simulink model "TA_Plant_Controller_Simulink"  (R2021a)
settings: Solver=ode45  StartTime=0.0  StopTime=1500  RelTol=1e-3  EnableMultiTasking=on
values from neighbouring files (symbols this model uses):
  Acu = 0    [TA_Plant_Controller_Param.m]
  Awa = 0.3    [TA_Plant_Controller_Param.m]
  Awi = 0    [TA_Plant_Controller_Param.m]
  d11 = ((6/11)^2)*d11    (= 74.3801652893)    [TA_Plant_Controller_Param.m]
  d22 = ((6/11)^2)*d22    (= 431.404958678)    [TA_Plant_Controller_Param.m]
  d33 = 10*((6/11)^2)*d33    (= 4314.04958678)    [TA_Plant_Controller_Param.m]
  d44 = ((6/11)^2)*d44    (= 2380.16528926)    [TA_Plant_Controller_Param.m]
  d55 = ((6/11)^2)*d55    (= 44628.0991736)    [TA_Plant_Controller_Param.m]
  d66 = ((6/11)^2)*d66    (= 2380.16528926)    [TA_Plant_Controller_Param.m]
  dp2 = ((6/11)^2)*dp2    (= 0)    [TA_Plant_Controller_Param.m]
  dp3 = 0    [TA_Plant_Controller_Param.m]
  dq2 = ((6/11)^2)*dq2    (= 0)    [TA_Plant_Controller_Param.m]
  dq3 = 0    [TA_Plant_Controller_Param.m]
  dr2 = ((6/11)^2)*dr2    (= 59.5041322314)    [TA_Plant_Controller_Param.m]
  dr3 = 0    [TA_Plant_Controller_Param.m]
  du2 = ((6/11)^2)*du2    (= 59.5041322314)    [TA_Plant_Controller_Param.m]
  du3 = 0    [TA_Plant_Controller_Param.m]
  dv2 = ((6/11)^2)*dv2    (= 273.748760331)    [TA_Plant_Controller_Param.m]
  dv3 = 0    [TA_Plant_Controller_Param.m]
  dw2 = ((6/11)^2)*dw2    (= 273.748760331)    [TA_Plant_Controller_Param.m]
  dw3 = 0    [TA_Plant_Controller_Param.m]
  g = 9.8    [TA_Plant_Controller_Param.m]
  intpitch = 0    [TA_Plant_Controller_Param.m]
  introll = 0    [TA_Plant_Controller_Param.m]
  intz = 0    [TA_Plant_Controller_Param.m]
  Kb = 1000    [TA_Plant_Controller_Param.m]
  kpitch = 50    [TA_Plant_Controller_Param.m]
  kroll = 1.5    [TA_Plant_Controller_Param.m]
  kuu = 1140    [TA_Plant_Controller_Param.m]
  kvr = 20000    [TA_Plant_Controller_Param.m]
  m11 = ((6/11)^2)*m11    (= 312.396694215)    [TA_Plant_Controller_Param.m]
  m22 = ((6/11)^2)*m22    (= 357.024793388)    [TA_Plant_Controller_Param.m]
  m33 = ((6/11)^2)*m33    (= 362.975206612)    [TA_Plant_Controller_Param.m]
  m44 = ((6/11)^2)*m44    (= 459.683676155)    [TA_Plant_Controller_Param.m]
  m55 = ((6/11)^2)*m55    (= 9595.04132231)    [TA_Plant_Controller_Param.m]
  m66 = ((6/11)^2)*m66    (= 9600.99173554)    [TA_Plant_Controller_Param.m]
  mode_gangguan = 1    [TA_Plant_Controller_Param.m]
  rho = 1025    [TA_Plant_Controller_Param.m]
  Ts = 0.05    [TA_Plant_Controller_Param.m]
  vol = ((6/11)^2)*6.6206    (= 1.96976528926)    [TA_Plant_Controller_Param.m]
undefined symbols (not defined in the file or in its folder): magnitude
libraries: mpclib x1, simulink x1
settings Model: Creator=farabialif  LastModifiedBy=billy
settings SolverCC: AlgebraicLoopSolver=TrustRegion
settings DataIOCC: LimitDataPoints=on  SaveFormat=Array  ReturnWorkspaceOutputs=off
settings OptimizationCC: LifeSpan=inf
settings DebuggingCC: SolverPrmCheckMsg=warning  SFUnexpectedBacktrackingDiag=warning  SFNoUnconditionalDefaultTransitionDiag=warning  SFExecutionAtInitializationDiag=none  SFMachineParentedDataDiag=warning  ArithmeticOperatorsInVariantConditions=warning
settings HardwareCC: ProdBitPerPointer=32  ProdBitPerSizeT=32  ProdBitPerPtrDiffT=32  ProdLargestAtomicFloat=None  ProdIntDivRoundTo=Undefined  ProdEndianess=Unspecified  ProdWordSize=32  ProdHWDeviceType=32-bit Generic
settings ModelReferenceCC: PropagateSignalLabelsOutOfModel=off
settings SFSimCC: SimUseLocalCustomCode=off  CustomCodeUndefinedFunction=UseInterfaceOnly
settings RTWCC: RTWUseLocalCustomCode=off
settings CodeAppCC: StateflowObjectComments=on
settings GRTTargetCC: TargetLangStandard=C89/C90 (ANSI)
settings ConfigComp: CovMetricSettings=dw  CovSaveCumulativeToWorkspaceVar=on  CovSaveSingleToWorkspaceVar=on  CovExternalEMLEnable=off  CovSFcnEnable=off

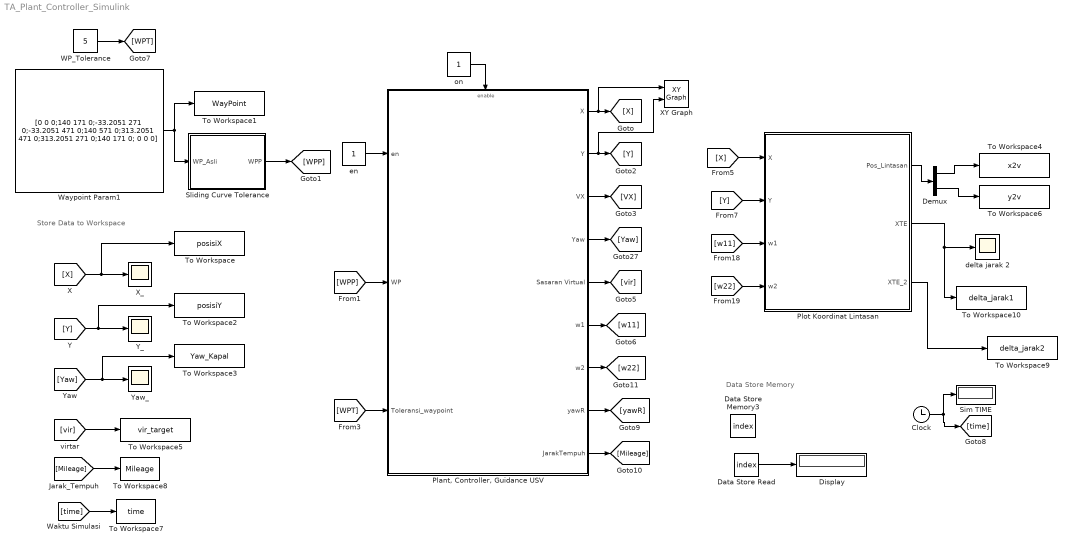
== system TA_Plant_Controller_Simulink ==
  note: Data Store Memory
  note: Store Data to Workspace
  Clock : Clock
  Data Store Memory3 : DataStoreMemory  DataStoreName=index  ReadBeforeWriteMsg=warning  WriteAfterWriteMsg=warning  WriteAfterReadMsg=warning  ShowAdditionalParam=off  OutDataTypeStr=int8  Dimensions=1
  Data Store Read : DataStoreRead  DataStoreName=index  IndexOptions=Index vector (dialog)  Indices=1  OutputSizes=1
  Demux : Demux  Outputs=2
  Display : Display
  "Plant, Controller, Guidance USV" : Subsystem
  Plot Koordinat Lintasan : MATLAB Function  TreatAsAtomicUnit=on
  Sim TIME : Display
  Sliding Curve Tolerance : MATLAB Function  TreatAsAtomicUnit=on
  To Workspace : ToWorkspace  VariableName=posisiX  SaveFormat=Timeseries  SampleTime=-1
  To Workspace1 : ToWorkspace  VariableName=WayPoint  SampleTime=-1
  To Workspace10 : ToWorkspace  VariableName=delta_jarak1  SaveFormat=Timeseries  SampleTime=-1
  To Workspace2 : ToWorkspace  VariableName=posisiY  SaveFormat=Timeseries  SampleTime=-1
  To Workspace3 : ToWorkspace  VariableName=Yaw_Kapal  SaveFormat=Timeseries  SampleTime=-1
  To Workspace4 : ToWorkspace  VariableName=x2v  SaveFormat=Timeseries  SampleTime=-1
  To Workspace5 : ToWorkspace  VariableName=vir_target  SaveFormat=Timeseries  SampleTime=-1
  To Workspace6 : ToWorkspace  VariableName=y2v  SaveFormat=Timeseries  SampleTime=-1
  To Workspace7 : ToWorkspace  VariableName=time  SaveFormat=Timeseries  SampleTime=-1
  To Workspace8 : ToWorkspace  VariableName=Mileage  SaveFormat=Timeseries  SampleTime=-1
  To Workspace9 : ToWorkspace  VariableName=delta_jarak2  SaveFormat=Timeseries  SampleTime=-1
  WP_Tolerance : Constant  Value=5
  Waypoint Param1 : Constant  Value=[0 0 0;140 171 0;-33.2051 271 0;-33.2051 471 0;140 571 0;313.2051 471 0;313.2051 271 0;140 171 0; 0 0 0]
  XY Graph : simulink/Sinks/XY Graph  xmin=-100  xmax=350  ymin=-20  ymax=600  st=-1
  X_ : Scope
  Y_ : Scope
  Yaw_ : Scope
  delta jarak 2 : Scope
  en : Constant
  on : Constant
  wires:
  on/1 -> "Plant, Controller, Guidance USV"/Enable
  en/1 -> "Plant, Controller, Guidance USV"/1("en ")
  WP_Tolerance/1 -> [WPT]
  [WPT] -> "Plant, Controller, Guidance USV"/3(Toleransi_waypoint)
  [Y] -> To Workspace2/1, Y_/1
  [X] -> To Workspace/1, X_/1
  [Yaw] -> To Workspace3/1, Yaw_/1
  [vir] -> To Workspace5/1
  Waypoint Param1/1 -> Sliding Curve Tolerance/1(WP_Asli), To Workspace1/1
  [WPP] -> "Plant, Controller, Guidance USV"/2(WP)
  "Plant, Controller, Guidance USV"/6(w1) -> [w11]
  "Plant, Controller, Guidance USV"/1(X) -> XY Graph/1, [X]
  "Plant, Controller, Guidance USV"/2(Y) -> XY Graph/2, [Y]
  "Plant, Controller, Guidance USV"/5(Sasaran Virtual) -> [vir]
  "Plant, Controller, Guidance USV"/4(Yaw) -> [Yaw]
  "Plant, Controller, Guidance USV"/7(w2) -> [w22]
  "Plant, Controller, Guidance USV"/3(VX) -> [VX]
  [X] -> Plot Koordinat Lintasan/1(X)
  [Y] -> Plot Koordinat Lintasan/2(Y)
  [w11] -> Plot Koordinat Lintasan/3(w1)
  [w22] -> Plot Koordinat Lintasan/4(w2)
  Clock/1 -> [time], Sim TIME/1
  "Plant, Controller, Guidance USV"/8(yawR) -> [yawR]
  "Plant, Controller, Guidance USV"/9(JarakTempuh) -> [Mileage]
  Data Store Read/1 -> Display/1
  Sliding Curve Tolerance/1(WPP) -> [WPP]
  Plot Koordinat Lintasan/1(Pos_Lintasan) -> Demux/1
  Demux/1 -> To Workspace4/1
  Demux/2 -> To Workspace6/1
  Plot Koordinat Lintasan/2(XTE) -> To Workspace10/1, delta jarak 2/1
  [Mileage] -> To Workspace8/1
  [time] -> To Workspace7/1
  Plot Koordinat Lintasan/3(XTE_2) -> To Workspace9/1

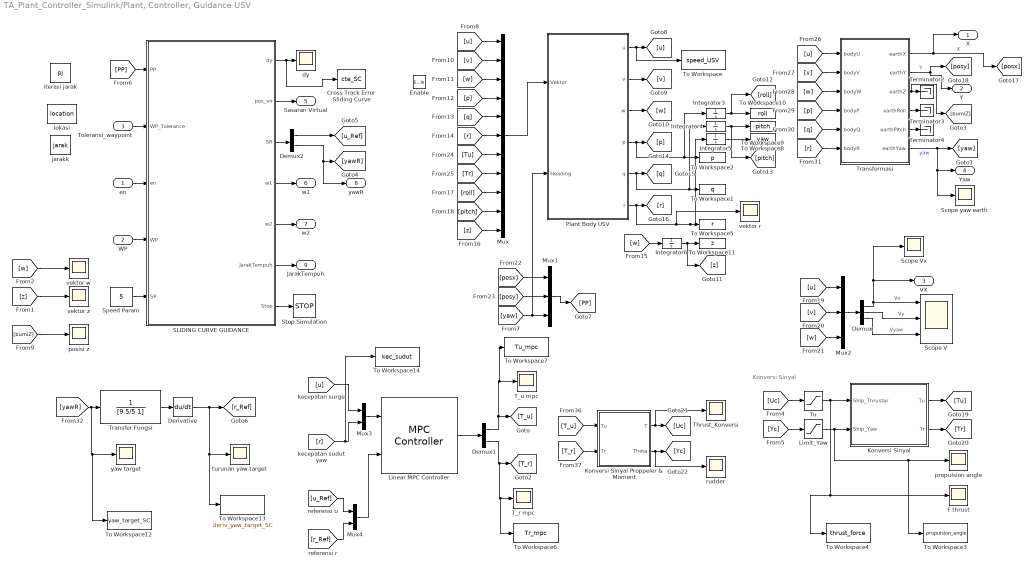
== system TA_Plant_Controller_Simulink/Plant, Controller, Guidance USV ==
  note: Konversi Sinyal
  "en " : Inport
  WP : Inport  Port=2
  Toleransi_waypoint : Inport  Port=3
  Enable : EnablePort
  Cross Track Error Sliding Curve : ToWorkspace  VariableName=cte_SC  SaveFormat=Timeseries  SampleTime=Ts
  Demux : Demux  Outputs=3
  Demux1 : Demux  Outputs=2
  Demux2 : Demux  Outputs=2
  Derivative : Derivative  CoefficientInTFapproximation=Ts
  F thrust : Scope
  Integrator3 : Integrator  InitialCondition=introll
  Integrator4 : Integrator  InitialCondition=intpitch
  Integrator5 : Integrator
  Integrator6 : Integrator  InitialCondition=intz
  Konversi Sinyal : MATLAB Function  TreatAsAtomicUnit=on
  Konversi Sinyal Proppeler & Moment : MATLAB Function  TreatAsAtomicUnit=on
  Limit_Yaw : Saturate  UpperLimit=1.0472  LowerLimit=-1.0472
  Linear MPC Controller : mpclib/MPC Controller  SCDEnableBlockLinearizationSpecification=on  mpcobj=mpc04  is_multiple=0  enable_value=0  return_u0=off  updateMPCinCallerWorkspace=on  md_inport=off  mv_inport=off  uref_inport=off  return_cost=off  return_mvseq=off  return_qpstatus=off  return_xseq=off  return_state=off  return_ovseq=off  state_inport=off  umin_inport=off  umax_inport=off  ymin_inport=off  ymax_inport=off  cc_inport=off  ywt_inport=off  uwt_inport=off  duwt_inport=off  rhoeps_inport=off  pm_inport=off  MaximumP=10  HorizonChoice=FixedHorizon  n_ts=0.05  n_p=25  n_mv=2  n_md=0  n_ud=0  n_mo=2  n_uo=0  BlockDataType=double  SampleTimeInherited=off  switch_inport=off
  Mux : Mux  Inputs=11
  Mux1 : Mux  Inputs=3
  Mux2 : Mux  Inputs=3
  Mux3 : Mux  Inputs=2
  Mux4 : Mux  Inputs=2
  Plant Body USV : Subsystem
  SLIDING CURVE GUIDANCE : MATLAB Function  TreatAsAtomicUnit=on
  Scope V : Scope  NumInputPorts=3
  Scope Vx : Scope
  Scope yaw earth : Scope
  Speed Param : Constant  Value=5
  Stop Simulation : Stop
  T_r mpc : Scope
  T_u mpc : Scope
  Terminator2 : Terminator
  Terminator3 : Terminator
  Terminator4 : Terminator
  Thrust_Konversi : Scope
  To Workspace : ToWorkspace  VariableName=speed_USV  SaveFormat=Timeseries  SampleTime=-1
  To Workspace1 : ToWorkspace  VariableName=q  SampleTime=-1
  To Workspace10 : ToWorkspace  VariableName=roll  SampleTime=-1
  To Workspace11 : ToWorkspace  VariableName=z  SampleTime=-1
  To Workspace12 : ToWorkspace  VariableName=yaw_target_SC  SaveFormat=Timeseries  SampleTime=-1
  To Workspace13 : ToWorkspace  VariableName=deriv_yaw_target_SC  SaveFormat=Timeseries  SampleTime=-1
  To Workspace14 : ToWorkspace  VariableName=kec_sudut  SaveFormat=Timeseries  SampleTime=-1
  To Workspace2 : ToWorkspace  VariableName=p  SampleTime=-1
  To Workspace3 : ToWorkspace  VariableName=propulsion_angle  SaveFormat=Timeseries  SampleTime=-1
  To Workspace4 : ToWorkspace  VariableName=thrust_force  SaveFormat=Timeseries  SampleTime=-1
  To Workspace5 : ToWorkspace  VariableName=r  SampleTime=-1
  To Workspace6 : ToWorkspace  VariableName=Tr_mpc  SaveFormat=Timeseries  SampleTime=-1
  To Workspace7 : ToWorkspace  VariableName=Tu_mpc  SaveFormat=Timeseries  SampleTime=-1
  To Workspace8 : ToWorkspace  VariableName=yaw  SampleTime=-1
  To Workspace9 : ToWorkspace  VariableName=pitch  SampleTime=-1
  Transfer Fungsi : TransferFcn  Denominator=[9.5/5 1]
  Transformasi : Subsystem
  Tu : Saturate  UpperLimit=10000  LowerLimit=0
  dy : Scope
  iterasi jarak : DataStoreMemory  DataStoreName=pj  ReadBeforeWriteMsg=warning  WriteAfterWriteMsg=warning  WriteAfterReadMsg=warning  InitialValue=1  ShowAdditionalParam=off  OutDataTypeStr=double  Dimensions=1
  jarakk : DataStoreMemory  DataStoreName=jarak  ReadBeforeWriteMsg=warning  WriteAfterWriteMsg=warning  WriteAfterReadMsg=warning  ShowAdditionalParam=off  OutDataTypeStr=double  Dimensions=1
  lokasi : DataStoreMemory  DataStoreName=location  ReadBeforeWriteMsg=warning  WriteAfterWriteMsg=warning  WriteAfterReadMsg=warning  ShowAdditionalParam=off  OutDataTypeStr=double  Dimensions=[2,2]
  posisi z : Scope
  propulsion angle : Scope
  rudder : Scope
  turunan yaw target : Scope
  vektor r : Scope
  vektor w : Scope
  vektor z : Scope
  yaw target : Scope
  X : Outport  VectorParamsAs1DForOutWhenUnconnected=off
  Y : Outport  Port=2  VectorParamsAs1DForOutWhenUnconnected=off
  VX : Outport  Port=3  VectorParamsAs1DForOutWhenUnconnected=off
  Yaw : Outport  Port=4  VectorParamsAs1DForOutWhenUnconnected=off
  Sasaran Virtual : Outport  Port=5  VectorParamsAs1DForOutWhenUnconnected=off
  w1 : Outport  Port=6  VectorParamsAs1DForOutWhenUnconnected=off
  w2 : Outport  Port=7  VectorParamsAs1DForOutWhenUnconnected=off
  yawR : Outport  Port=8  VectorParamsAs1DForOutWhenUnconnected=off
  JarakTempuh : Outport  Port=9  VectorParamsAs1DForOutWhenUnconnected=off
  wires:
  [v] -> Mux/2
  Mux/1 -> Plant Body USV/1(Vektor)
  Toleransi_waypoint/1 -> SLIDING CURVE GUIDANCE/2(WP_Tolerance)
  Demux2/2 -> yawR/1, [yawR]
  [bumiZ] -> posisi z/1
  Limit_Yaw/1 -> Konversi Sinyal/2(Ship_Yaw), propulsion angle/1, To Workspace3/1
  Plant Body USV/4(p) -> To Workspace2/1, Integrator3/1, [p]
  SLIDING CURVE GUIDANCE/1(dy) -> Cross Track Error Sliding Curve/1, dy/1
  SLIDING CURVE GUIDANCE/2(pos_vir) -> Sasaran Virtual/1
  Transformasi/3(earthZ) -> Terminator2/1, [bumiZ]
  Transformasi/1(earthX) -> X/1, [posx]  "X"
  Plant Body USV/5(q) -> To Workspace1/1, Integrator4/1, [q]
  [q] -> Mux/5
  Speed Param/1 -> SLIDING CURVE GUIDANCE/5(SP)
  Plant Body USV/2(v) -> [v]
  Demux/3 -> Scope V/3  "Vyaw"
  WP/1 -> SLIDING CURVE GUIDANCE/4(WP)
  [w] -> vektor w/1
  [r] -> Mux/6
  SLIDING CURVE GUIDANCE/3(SR) -> Demux2/1
  [u] -> Mux2/1
  Plant Body USV/6(r) -> vektor r/1, To Workspace5/1, Integrator5/1, [r]
  SLIDING CURVE GUIDANCE/5(w2) -> w2/1
  Transformasi/2(earthY) -> Y/1, [posy]  "Y"
  [roll] -> Mux/9
  "en "/1 -> SLIDING CURVE GUIDANCE/3(en)
  [Tu] -> Mux/7
  Konversi Sinyal/2(Tr) -> [Tr]
  Plant Body USV/1(u) -> To Workspace/1, [u]
  Integrator3/1 -> [roll], To Workspace10/1
  [u] -> Transformasi/1(bodyU)
  [posx] -> Mux1/1
  [u] -> Mux/1
  [pitch] -> Mux/10
  Transformasi/5(earthPitch) -> Terminator4/1
  Transformasi/6(earthYaw) -> Scope yaw earth/1, Yaw/1, [yaw]  "yaw"
  [q] -> Transformasi/5(bodyQ)
  [posy] -> Mux1/2
  [w] -> Mux2/3
  [z] -> vektor z/1
  Integrator4/1 -> To Workspace9/1, [pitch]
  SLIDING CURVE GUIDANCE/4(w1) -> w1/1
  [v] -> Transformasi/2(bodyV)
  Demux/2 -> Scope V/2  "Vy"
  [r] -> Transformasi/6(bodyR)
  [p] -> Mux/4
  [yaw] -> Mux1/3, Plant Body USV/2(Heading)
  [PP] -> SLIDING CURVE GUIDANCE/1(PP)
  Demux/1 -> VX/1, Scope Vx/1, Scope V/1  "Vx"
  SLIDING CURVE GUIDANCE/7(Stop) -> Stop Simulation/1
  Integrator5/1 -> To Workspace8/1
  [Tr] -> Mux/8
  [w] -> Integrator6/1
  Mux1/1 -> [PP]
  [z] -> Mux/11
  [w] -> Mux/3
  Plant Body USV/3(w) -> [w]
  Integrator6/1 -> [z], To Workspace11/1
  [p] -> Transformasi/4(bodyP)
  [w] -> Transformasi/3(bodyW)
  Transformasi/4(earthRoll) -> Terminator3/1
  Mux2/1 -> Demux/1
  [v] -> Mux2/2
  Konversi Sinyal/1(Tu) -> [Tu]
  Tu/1 -> Konversi Sinyal/1(Ship_Thruster), F thrust/1, To Workspace4/1
  [Yc] -> Limit_Yaw/1
  [Uc] -> Tu/1
  Demux2/1 -> [u_Ref]
  SLIDING CURVE GUIDANCE/6(JarakTempuh) -> JarakTempuh/1
  [r] -> To Workspace14/1, Mux3/2
  Mux3/1 -> Linear MPC Controller/1
  Mux4/1 -> Linear MPC Controller/2
  [u_Ref] -> Mux4/1
  [r_Ref] -> Mux4/2
  Linear MPC Controller/1 -> Demux1/1
  [yawR] -> To Workspace12/1, yaw target/1, Transfer Fungsi/1
  [T_u] -> Konversi Sinyal Proppeler & Moment/1(Tu)
  [T_r] -> Konversi Sinyal Proppeler & Moment/2(Tr)
  Transfer Fungsi/1 -> Derivative/1
  Demux1/1 -> To Workspace7/1, T_u mpc/1, [T_u]
  Demux1/2 -> To Workspace6/1, T_r mpc/1, [T_r]
  Konversi Sinyal Proppeler & Moment/1(T) -> Thrust_Konversi/1, [Uc]
  Konversi Sinyal Proppeler & Moment/2(Theta) -> rudder/1, [Yc]
  Derivative/1 -> To Workspace13/1, turunan yaw target/1, [r_Ref]
  [u] -> Mux3/1

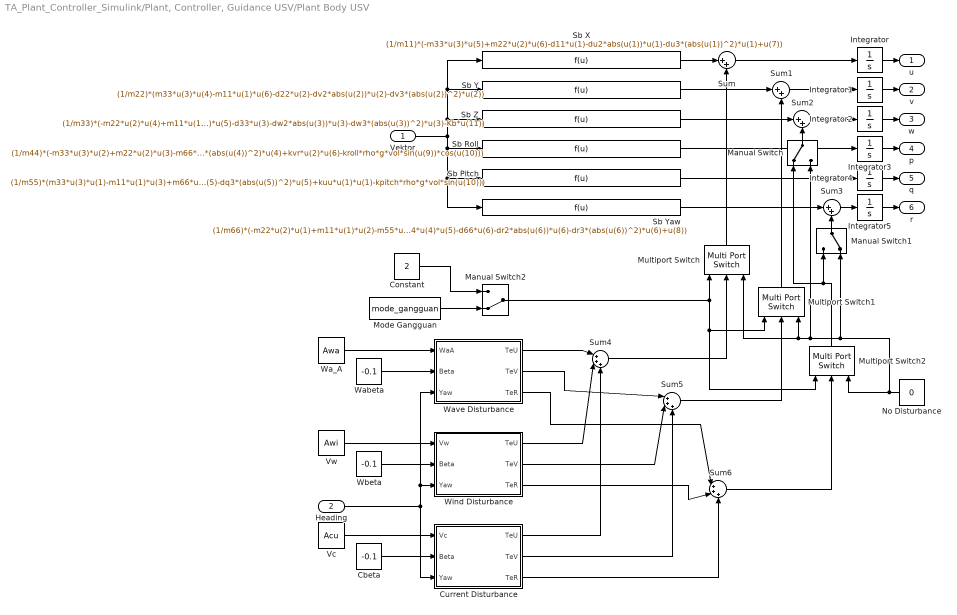
== system TA_Plant_Controller_Simulink/Plant, Controller, Guidance USV/Plant Body USV ==
  Vektor : Inport
  Heading : Inport  Port=2
  Cbeta : Constant  Value=-0.1
  Constant : Constant  Value=2
  Current Disturbance : Subsystem
  Integrator{,1..5} (6 alike) : Integrator
  Manual Switch : ManualSwitch
  Manual Switch1 : ManualSwitch  CurrentSetting=0
  Manual Switch2 : ManualSwitch  CurrentSetting=0
  Mode Gangguan : Constant  Value=mode_gangguan
  Multiport Switch : MultiPortSwitch  Inputs=2
  Multiport Switch1 : MultiPortSwitch  Inputs=2
  Multiport Switch2 : MultiPortSwitch  Inputs=2
  No Disturbance : Constant  Value=0
  Sb Pitch : Fcn  Expr=(1/m55)*(m33*u(3)*u(1)-m11*u(1)*u(3)+m66*u(6)*u(4)-m44*u(4)*u(6)-d55*u(5)-dq2*abs(u(5))*u(5)-dq3*(abs(u(5))^2)*u(5)+kuu*u(1)*u(1)-kpitch*rho*g*vol*sin(u(10)))
  Sb Roll : Fcn  Expr=(1/m44)*(-m33*u(3)*u(2)+m22*u(2)*u(3)-m66*u(6)*u(5)+m55*u(5)*u(6)-d44*u(4)-dp2*abs(u(4))*u(4)-dp3*(abs(u(4))^2)*u(4)+kvr*u(2)*u(6)-kroll*rho*g*vol*sin(u(9))*cos(u(10)))
  Sb X : Fcn  Expr=(1/m11)*(-m33*u(3)*u(5)+m22*u(2)*u(6)-d11*u(1)-du2*abs(u(1))*u(1)-du3*(abs(u(1))^2)*u(1)+u(7))
  Sb Y : Fcn  Expr=(1/m22)*(m33*u(3)*u(4)-m11*u(1)*u(6)-d22*u(2)-dv2*abs(u(2))*u(2)-dv3*(abs(u(2))^2)*u(2))
  Sb Yaw : Fcn  Expr=(1/m66)*(-m22*u(2)*u(1)+m11*u(1)*u(2)-m55*u(5)*u(4)+m44*u(4)*u(5)-d66*u(6)-dr2*abs(u(6))*u(6)-dr3*(abs(u(6))^2)*u(6)+u(8))
  Sb Z : Fcn  Expr=(1/m33)*(-m22*u(2)*u(4)+m11*u(1)*u(5)-d33*u(3)-dw2*abs(u(3))*u(3)-dw3*(abs(u(3))^2)*u(3)-Kb*u(11))
  Sum{,1..3} (4 alike) : Sum  Inputs=|++
  Sum4 : Sum  Inputs=|+++
  Sum5 : Sum  Inputs=|+++
  Sum6 : Sum  Inputs=|+++
  Vc : Constant  Value=Acu
  Vw : Constant  Value=Awi
  Wa_A : Constant  Value=Awa
  "Wabeta " : Constant  Value=-0.1
  Wave Disturbance : Subsystem
  Wbeta : Constant  Value=-0.1
  Wind Disturbance : Subsystem
  u : Outport  VectorParamsAs1DForOutWhenUnconnected=off
  v : Outport  Port=2  VectorParamsAs1DForOutWhenUnconnected=off
  w : Outport  Port=3  VectorParamsAs1DForOutWhenUnconnected=off
  p : Outport  Port=4  VectorParamsAs1DForOutWhenUnconnected=off
  q : Outport  Port=5  VectorParamsAs1DForOutWhenUnconnected=off
  r : Outport  Port=6  VectorParamsAs1DForOutWhenUnconnected=off
  wires:
  Vektor/1 -> Sb Z/1, Sb Y/1, Sb X/1, Sb Yaw/1, Sb Pitch/1, Sb Roll/1
  Sb Roll/1 -> Integrator3/1
  Sb Pitch/1 -> Integrator4/1
  Integrator/1 -> u/1
  Integrator1/1 -> v/1
  Integrator2/1 -> w/1
  Integrator3/1 -> p/1
  Integrator4/1 -> q/1
  Integrator5/1 -> r/1
  Sb X/1 -> Sum/1
  Sum/1 -> Integrator/1
  Sum1/1 -> Integrator1/1
  Sb Y/1 -> Sum1/1
  Multiport Switch/1 -> Sum/2
  No Disturbance/1 -> Multiport Switch2/3, Manual Switch1/2, Manual Switch/2, Multiport Switch1/3, Multiport Switch/3
  Multiport Switch2/1 -> Manual Switch1/1, Manual Switch/1
  Wind Disturbance/1(TeU) -> Sum4/2
  Wave Disturbance/1(TeU) -> Sum4/1
  Multiport Switch1/1 -> Sum1/2
  Manual Switch2/1 -> Multiport Switch2/1, Multiport Switch1/1, Multiport Switch/1
  Sum5/1 -> Multiport Switch1/2
  Sum4/1 -> Multiport Switch/2
  Sum6/1 -> Multiport Switch2/2
  Heading/1 -> Wave Disturbance/3(Yaw), Wind Disturbance/3(Yaw), Current Disturbance/3(Yaw)
  Vw/1 -> Wind Disturbance/1(Vw)
  Wind Disturbance/3(TeR) -> Sum6/2
  Wave Disturbance/2(TeV) -> Sum5/1
  Cbeta/1 -> Current Disturbance/2(Beta)
  Wa_A/1 -> Wave Disturbance/1(WaA)
  Wave Disturbance/3(TeR) -> Sum6/1
  Vc/1 -> Current Disturbance/1(Vc)
  Current Disturbance/1(TeU) -> Sum4/3
  Wbeta/1 -> Wind Disturbance/2(Beta)
  Wind Disturbance/2(TeV) -> Sum5/2
  "Wabeta "/1 -> Wave Disturbance/2(Beta)
  Current Disturbance/3(TeR) -> Sum6/3
  Current Disturbance/2(TeV) -> Sum5/3
  Sum2/1 -> Integrator2/1
  Sb Z/1 -> Sum2/1
  Manual Switch/1 -> Sum2/2
  Mode Gangguan/1 -> Manual Switch2/2
  Constant/1 -> Manual Switch2/1
  Sum3/1 -> Integrator5/1
  Sb Yaw/1 -> Sum3/1
  Manual Switch1/1 -> Sum3/2

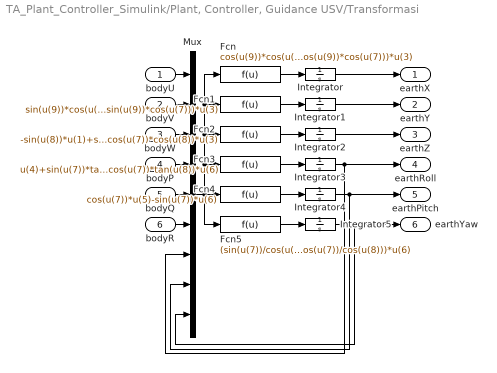
== system TA_Plant_Controller_Simulink/Plant, Controller, Guidance USV/Transformasi ==
  bodyU : Inport
  bodyV : Inport  Port=2
  bodyW : Inport  Port=3
  bodyP : Inport  Port=4
  bodyQ : Inport  Port=5
  bodyR : Inport  Port=6
  Fcn : Fcn  Expr=cos(u(9))*cos(u(8))*u(1)+(-sin(u(9))*cos(u(7))+sin(u(7))*sin(u(8))*cos(u(9)))*u(2)+(sin(u(9))*sin(u(7))+sin(u(8))*cos(u(9))*cos(u(7)))*u(3)
  Fcn1 : Fcn  Expr=sin(u(9))*cos(u(8))*u(1)+(cos(u(9))*cos(u(7))+sin(u(7))*sin(u(8))*sin(u(9)))*u(2)+(-cos(u(9))*sin(u(7))+sin(u(8))*sin(u(9))*cos(u(7)))*u(3)
  Fcn2 : Fcn  Expr=-sin(u(8))*u(1)+sin(u(7))*cos(u(8))*u(2)+cos(u(7))*cos(u(8))*u(3)
  Fcn3 : Fcn  Expr=u(4)+sin(u(7))*tan(u(8))*u(5)+cos(u(7))*tan(u(8))*u(6)
  Fcn4 : Fcn  Expr=cos(u(7))*u(5)-sin(u(7))*u(6)
  Fcn5 : Fcn  Expr=(sin(u(7))/cos(u(8)))*u(5)+(cos(u(7))/cos(u(8)))*u(6)
  Integrator{,1..5} (6 alike) : Integrator
  Mux : Mux  Inputs=9
  earthX : Outport
  earthY : Outport  Port=2
  earthZ : Outport  Port=3
  earthRoll : Outport  Port=4
  earthPitch : Outport  Port=5
  earthYaw : Outport  Port=6
  wires:
  bodyU/1 -> Mux/1
  bodyV/1 -> Mux/2
  bodyW/1 -> Mux/3
  bodyP/1 -> Mux/4
  bodyQ/1 -> Mux/5
  bodyR/1 -> Mux/6
  Mux/1 -> Fcn5/1, Fcn2/1, Fcn1/1, Fcn/1, Fcn3/1, Fcn4/1
  Fcn/1 -> Integrator/1
  Fcn5/1 -> Integrator5/1
  Fcn4/1 -> Integrator4/1
  Fcn1/1 -> Integrator1/1
  Fcn2/1 -> Integrator2/1
  Fcn3/1 -> Integrator3/1
  Integrator/1 -> earthX/1
  Integrator1/1 -> earthY/1
  Integrator4/1 -> earthPitch/1, Mux/8
  Integrator3/1 -> Mux/7, earthRoll/1
  Integrator2/1 -> earthZ/1
  Integrator5/1 -> earthYaw/1, Mux/9

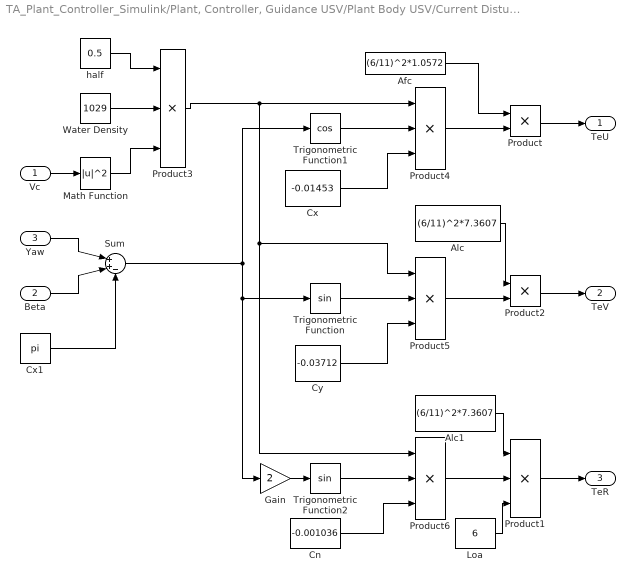
== system TA_Plant_Controller_Simulink/Plant, Controller, Guidance USV/Plant Body USV/Current Disturbance ==
  Vc : Inport
  Beta : Inport  Port=2
  Yaw : Inport  Port=3
  Afc : Constant  Value=(6/11)^2*1.0572
  Alc : Constant  Value=(6/11)^2*7.3607
  Alc1 : Constant  Value=(6/11)^2*7.3607
  Cn : Constant  Value=-0.001036
  Cx : Constant  Value=-0.01453
  Cx1 : Constant  Value=pi
  Cy : Constant  Value=-0.03712
  Gain : Gain  Gain=2
  Loa : Constant  Value=6
  Math Function : Math  Operator=magnitude^2  SignedPower=on  SaturateOnIntegerOverflow=on
  Product : Product
  Product{1,3..6} (5 alike) : Product  Inputs=3
  Product2 : Product
  Sum : Sum  Inputs=|++-
  Trigonometric Function : Trigonometry
  Trigonometric Function1 : Trigonometry  Operator=cos
  Trigonometric Function2 : Trigonometry
  Water Density : Constant  Value=1029
  half : Constant  Value=0.5
  TeU : Outport  VectorParamsAs1DForOutWhenUnconnected=off
  TeV : Outport  Port=2  VectorParamsAs1DForOutWhenUnconnected=off
  TeR : Outport  Port=3  VectorParamsAs1DForOutWhenUnconnected=off
  wires:
  Vc/1 -> Math Function/1
  Product/1 -> TeU/1
  Afc/1 -> Product/1
  Product2/1 -> TeV/1
  Alc/1 -> Product2/1
  Product1/1 -> TeR/1
  Alc1/1 -> Product1/1
  Loa/1 -> Product1/3
  Yaw/1 -> Sum/1
  Beta/1 -> Sum/2
  Cx1/1 -> Sum/3
  Water Density/1 -> Product3/2
  Math Function/1 -> Product3/3
  half/1 -> Product3/1
  Product4/1 -> Product/2
  Trigonometric Function1/1 -> Product4/2
  Cx/1 -> Product4/3
  Sum/1 -> Trigonometric Function1/1, Gain/1, Trigonometric Function/1
  Product3/1 -> Product6/1, Product5/1, Product4/1
  Product5/1 -> Product2/2
  Trigonometric Function/1 -> Product5/2
  Cy/1 -> Product5/3
  Product6/1 -> Product1/2
  Trigonometric Function2/1 -> Product6/2
  Cn/1 -> Product6/3
  Gain/1 -> Trigonometric Function2/1

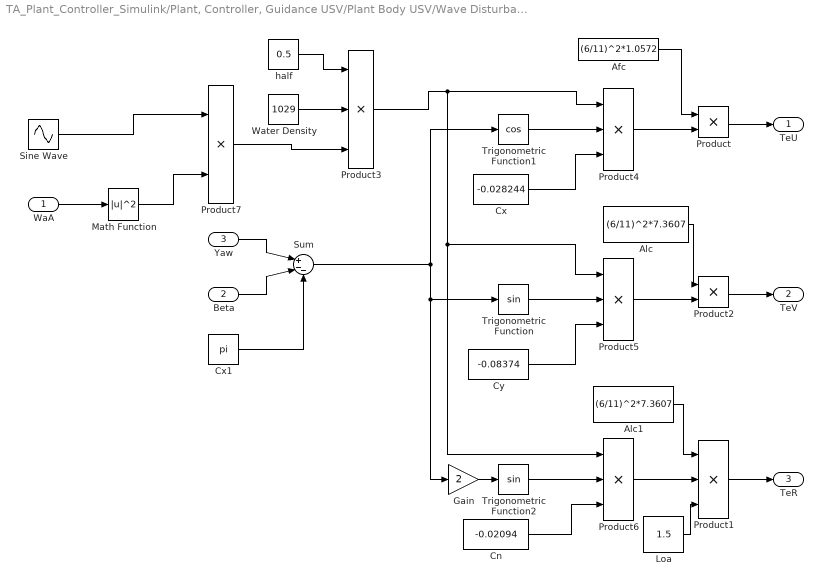
== system TA_Plant_Controller_Simulink/Plant, Controller, Guidance USV/Plant Body USV/Wave Disturbance ==
  WaA : Inport
  Beta : Inport  Port=2
  Yaw : Inport  Port=3
  Afc : Constant  Value=(6/11)^2*1.0572
  Alc : Constant  Value=(6/11)^2*7.3607
  Alc1 : Constant  Value=(6/11)^2*7.3607
  Cn : Constant  Value=-0.02094
  Cx : Constant  Value=-0.028244
  Cx1 : Constant  Value=pi
  Cy : Constant  Value=-0.08374
  Gain : Gain  Gain=2
  Loa : Constant  Value=1.5
  Math Function : Math  Operator=magnitude^2  SignedPower=on  SaturateOnIntegerOverflow=on
  Product : Product
  Product{1,3..6} (5 alike) : Product  Inputs=3
  Product2 : Product
  Product7 : Product
  Sine Wave : Sin  Frequency=0.08  SampleTime=0
  Sum : Sum  Inputs=|+--
  Trigonometric Function : Trigonometry
  Trigonometric Function1 : Trigonometry  Operator=cos
  Trigonometric Function2 : Trigonometry
  Water Density : Constant  Value=1029
  half : Constant  Value=0.5
  TeU : Outport  VectorParamsAs1DForOutWhenUnconnected=off
  TeV : Outport  Port=2  VectorParamsAs1DForOutWhenUnconnected=off
  TeR : Outport  Port=3  VectorParamsAs1DForOutWhenUnconnected=off
  wires:
  Product/1 -> TeU/1
  Afc/1 -> Product/1
  Product2/1 -> TeV/1
  Alc/1 -> Product2/1
  Product1/1 -> TeR/1
  Loa/1 -> Product1/3
  Yaw/1 -> Sum/1
  Beta/1 -> Sum/2
  Cx1/1 -> Sum/3
  Water Density/1 -> Product3/2
  half/1 -> Product3/1
  Product4/1 -> Product/2
  Trigonometric Function1/1 -> Product4/2
  Cx/1 -> Product4/3
  Sum/1 -> Trigonometric Function1/1, Gain/1, Trigonometric Function/1
  Product3/1 -> Product6/1, Product5/1, Product4/1
  Product5/1 -> Product2/2
  Trigonometric Function/1 -> Product5/2
  Cy/1 -> Product5/3
  Product6/1 -> Product1/2
  Trigonometric Function2/1 -> Product6/2
  Cn/1 -> Product6/3
  Gain/1 -> Trigonometric Function2/1
  Sine Wave/1 -> Product7/1
  WaA/1 -> Math Function/1
  Math Function/1 -> Product7/2
  Product7/1 -> Product3/3
  Alc1/1 -> Product1/1

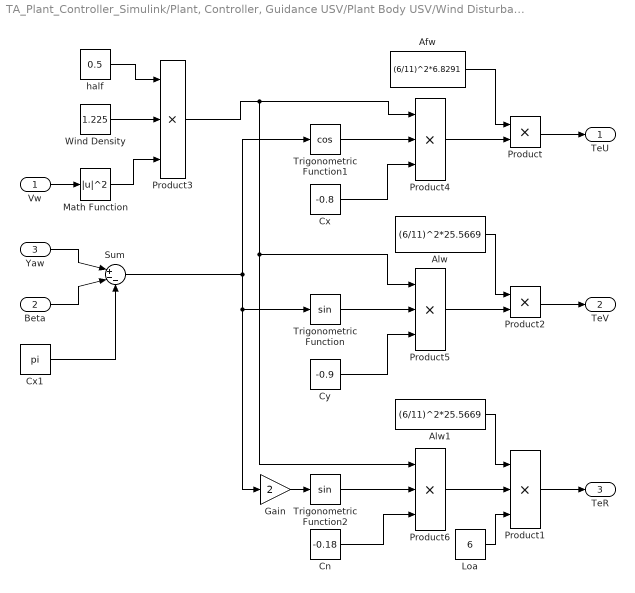
== system TA_Plant_Controller_Simulink/Plant, Controller, Guidance USV/Plant Body USV/Wind Disturbance ==
  Vw : Inport
  Beta : Inport  Port=2
  Yaw : Inport  Port=3
  Afw : Constant  Value=(6/11)^2*6.8291
  Alw : Constant  Value=(6/11)^2*25.5669
  Alw1 : Constant  Value=(6/11)^2*25.5669
  Cn : Constant  Value=-0.18
  Cx : Constant  Value=-0.8
  Cx1 : Constant  Value=pi
  Cy : Constant  Value=-0.9
  Gain : Gain  Gain=2
  Loa : Constant  Value=6
  Math Function : Math  Operator=magnitude^2  SignedPower=on  SaturateOnIntegerOverflow=on
  Product : Product
  Product{1,3..6} (5 alike) : Product  Inputs=3
  Product2 : Product
  Sum : Sum  Inputs=|+--
  Trigonometric Function : Trigonometry
  Trigonometric Function1 : Trigonometry  Operator=cos
  Trigonometric Function2 : Trigonometry
  Wind Density : Constant  Value=1.225
  half : Constant  Value=0.5
  TeU : Outport  VectorParamsAs1DForOutWhenUnconnected=off
  TeV : Outport  Port=2  VectorParamsAs1DForOutWhenUnconnected=off
  TeR : Outport  Port=3  VectorParamsAs1DForOutWhenUnconnected=off
  wires:
  Vw/1 -> Math Function/1
  Product/1 -> TeU/1
  Afw/1 -> Product/1
  Product2/1 -> TeV/1
  Alw/1 -> Product2/1
  Product1/1 -> TeR/1
  Alw1/1 -> Product1/1
  Loa/1 -> Product1/3
  Yaw/1 -> Sum/1
  Beta/1 -> Sum/2
  Cx1/1 -> Sum/3
  Wind Density/1 -> Product3/2
  Math Function/1 -> Product3/3
  half/1 -> Product3/1
  Product4/1 -> Product/2
  Trigonometric Function1/1 -> Product4/2
  Cx/1 -> Product4/3
  Sum/1 -> Trigonometric Function1/1, Gain/1, Trigonometric Function/1
  Product3/1 -> Product6/1, Product5/1, Product4/1
  Product5/1 -> Product2/2
  Trigonometric Function/1 -> Product5/2
  Cy/1 -> Product5/3
  Product6/1 -> Product1/2
  Trigonometric Function2/1 -> Product6/2
  Cn/1 -> Product6/3
  Gain/1 -> Trigonometric Function2/1

== matlab function TA_Plant_Controller_Simulink/Plot Koordinat Lintasan ==
  data: X input; Y input; w1 input; w2 input; Pos_Lintasan output; XTE output; XTE_2 output
function [Pos_Lintasan,XTE, XTE_2]  = Koordinat_Lintasan(X, Y, w1, w2)
% Deskripsi I?O
% Input
% X, Y: Posisi Kapal
% w1, w2: Waypoint

% Output
% Pos_Lintasan: Koordinat Lintasan menggunakan rumus : [x2v, y2v]
% cte : Cross Track Error [delta_jarak delta_jarak2]

% Transformasi Koordinat dan Simpan data X Y USV
% Ini versi tanpa di transformasi
XY = [X Y] % matriks posisi
Xusv=XY(1); % x 
Yusv=XY(2); % y
a = Xusv;
b = Yusv;

% titik lintasan awal atau sebelum (yang dituju sebelum)
w1_x = w1(1);
w1_y = w1(2);
%titik lintasan sesudah (yang dituju sesudah)
w2_x = w2(1);
w2_y = w2(2);

% persamaan garis lurus antar dua titik 
% (y-y1)/(y2-y1)=(x-x1)/(x2-x1) => px+qy+r=0
p = w2_y-w1_y;
q = w1_x-w2_x;
r = (w1_y-w2_y)*w1_x+(w2_x-w1_x)*w1_y

% koordinat lintasan referensinya berdasarkan persamaan garis lurus
x2v = (a*q^2-b*p*q-p*r)/(p^2+q^2);
y2v = ((q/p)*(a*q^2-b*p*q-p*r)/(p^2+q^2))+(b*p-a*q)/(p);

Pos_Lintasan = [x2v y2v];
% Cross Track Error Antar Lintasan
% jarak lintasan dengan usv
% jarak lintasan menggunakan rumus jadi
delta_jarak1 = (abs(p*a+q*b+r)/sqrt(p^2+q^2));
delta_jarak2 = sqrt((x2v-a).^2+(y2v-b).^2);
%Cross_Track_Error = [delta_jarak delta_jarak2];
XTE = delta_jarak1;
XTE_2 = delta_jarak2;
end

== matlab function TA_Plant_Controller_Simulink/Plant, Controller, Guidance USV/Konversi Sinyal ==
  data: Ship_Thruster input; Tu output; Ship_Yaw input; Tr output
function [Tu,Tr] = CV(Ship_Thruster,Ship_Yaw)
Tu=Ship_Thruster*cos(Ship_Yaw);
Tr=Ship_Thruster*sin(Ship_Yaw);
end

== matlab function TA_Plant_Controller_Simulink/Plant, Controller, Guidance USV/Konversi Sinyal Proppeler & Moment ==
  data: Tu input; T output; Tr input; Theta output
function [T, Theta]= CTuTr (Tu,Tr)
T_max= 2000;
Tr_max = 3464.102;
Theta = atan2(Tr,Tu);
Theta_max = 1.0472;
p = cos(Theta);
if p==0
    T = T_max;
else
    T=Tu/p;
end
%if Theta>Theta_max
%    Theta = Theta_max;
%end
%if Tr>Tr_max
%   Tr = Tr_max; 
%end
%if T>T_max
%    T=T_max;
%end
end

== matlab function TA_Plant_Controller_Simulink/Sliding Curve Tolerance ==
  data: WP_Asli input; WPP output
function WPP  = SCToleranvce(WP_Asli)
WP =WP_Asli;
WPP = [WP;-32 -32 0];
end

== matlab function TA_Plant_Controller_Simulink/Plant, Controller, Guidance USV/SLIDING CURVE GUIDANCE ==
  settings: updateMethod=DISCRETE
  data: PP input size=3; WP_Tolerance input; en input; dy output; pos_vir output; SR output; WP input; SP input; w1 output; w2 output; JarakTempuh output; Stop output; pj data_store_memory; location data_store_memory; jarak data_store_memory; index data_store_memory
function [dy, pos_vir, SR, w1, w2, JarakTempuh, Stop]= Waypoint_Planner(PP, WP_Tolerance, en, WP, SP)
global index pj jarak location
%Penjelasan variabel
%Variabel Input
%   PP: Present locationition     : [x,y]
%   WP_Tolerance: Toleransi       : [constant]
%   WP: Waypoint                  : [x_target,y_target,Toleransi_waypoint]
%   SP: Speed Parameter           : [Speed_max,waktu_menuju_target]
%   en: Enable                    : [Enable_bit]
%   delta_SC: Delta Sliding Curve : [delta]

%Variabel Output
%   dy: Sliding Curve Cross Track Error
%   pos_vir : Sasaran virtual     : [x_vir y_vir]
%   SR: Ship Refference           : [Speed_Target Yaw_Target]
%   w1, w2: Waypoint Sebelum dan Setelah :[w1_x w1_y], [w2_x w2_y]
%   JarakTempuh : Jarak Tempuh Kapal : jarak
%   Stop : Stop Simulasi          : STOP
%   ST: Status                    : [bit_status]

% Deklarasi Variable Input
% Input X, Y, dan Yaw
x = PP(1);
y = PP(2);
yaw = PP(3);
% SP
Speed_max = SP;
% WP_Tolerance
toleransi_waypoint= WP_Tolerance;
% Enable_bit
Enable_bit = en;
% Delta minimum sliding curve
delta=15; %delta=20 
A=index; % Pergantian index waypoint

%%SLIDING CURVE GUIDANCE 
% SLIDING STRAIGHT LINE
% Waypoint P
%w1 = posisi sebelum
%w2 = posisi saat ini/sesudah
w2_x=WP(A+2,1); % x target sesudah
w1_x=WP(A+1,1); %wpts1 - x target sebelum
w2_y=WP(A+2,2); % y target sesudah
w1_y=WP(A+1,2); %wpts1 - y target sebelum

w1 = [w1_x w1_y];
w2 = [w2_x w2_y];

%Transformasi acuan bumi ke acuan kapal
length_x_sebelum=w2_x-w1_x;
length_y_sebelum=w2_y-w1_y;

% Sliding Yaw
R_uy = sqrt((w1_x-x)^2 + (w1_y-y)^2);   %Ru untuk yaw 
thetay = atan2((w2_y-w1_y),(w2_x-w1_x));%Theta bidang x-y
% Jarak dan sudut antara Wi dan Wi+1
theta_uy = atan2((y-w1_y),(x-w1_x));    %thetau x-y
betay = thetay-theta_uy;
% Sudut antara Wi dengan posisi sekarang serta sudut beta
dy = R_uy*sin(betay);
Ry = sqrt(R_uy^2-(R_uy*sin(betay))^2);  %Beta x-y
% Update dari posisi sasaran atau virtual target
x_target = w1_x+(Ry+delta)*cos(thetay); 
y_target = w1_y+(Ry+delta)*sin(thetay);
% Posisi X dan Y virtual untuk Plot
x_vir = x_target;
y_vir = y_target;
pos_vir = [x_vir y_vir]; 
% sudut arah target USV untuk mengejar sasaran virtual
Yaw_Target = atan2((y_target-y),(x_target-x)); %DESIRED YAW

%Transformasi acuan bumi ke acuan kapal
length_x=w2_x-x_target;
length_y=w2_y-y_target;

%menghitung JARAK TEMPUH >>>>>>>>>>>>>>>>>>>>>>>
dist=0;
if pj==1
location(1,:)=[x y];
elseif pj==2
location(2,:)=[x y];
elseif pj>=3
location(1,:)=location(2,:);
location(2,:)=[x y];
end
dist=sqrt((location(2,2)-location(1,2))^2+(location(2,1)-location(1,1))^2);
jarak=jarak+dist;
JarakTempuh=jarak;
pj=pj+1;

wpfinal_x=WP(end-1,1);
wpfinal_y=WP(end-1,2);
Lx=wpfinal_x-x;
Ly=wpfinal_y-y;
length_resultan=sqrt(Lx^2+Ly^2);
%length_resultan_constant=sqrt(length_x_sebelum^2+length_y_sebelum^2);
Speed_Target = Speed_max;

% Ketika WP akhir di 8
if  A >=6 && length_resultan<=(toleransi_waypoint+1)
    Stop=1;
else
    Stop=0;
end

%menyatakan status planner
if abs(length_x)<=toleransi_waypoint && abs(length_y)<=toleransi_waypoint
    bit_status=1;
    Enable_Bit=0;
    index=index+1;
    A=index;
    %Speed_Target=0.1*Speed_max;
else
    bit_status=0;
end

if Enable_bit==1
% menulis Variabel Output
    SR=[Speed_Target Yaw_Target];
% DW=[length_resultan length_x length_y];
    ST=bit_status;
else
% menulis Variabel Output
    SR=[0 0]; %memberhentikan kontroller kapal
% DW=[length_resultan length_x length_y];
    ST=bit_status;
end
